simulink model "launch_sim"  (R2019a)
settings: Solver=ode4  StartTime=0.0  StopTime=20  FixedStep=.0001  RelTol=1e-3
values from neighbouring files (symbols this model uses):
  Cd = .51    (= 0.51)    [load_constants.m]
  diameter = 0.156337    [load_constants.m]
  padLat = 40.2    [load_constants.m]
  padLong = 76.8    [load_constants.m]
  propWeight = 1.2700    (= 1.27)    [motor.m]
  rocketMass = 15.51286 - totalWeight    [load_constants.m]
  thrust = thrustData(:,2)    [motor.m]
  thrustTime = thrustData(:,1)    [motor.m]
  totalImpulse = 2856.1    [motor.m]
  totalWeight = propWeight + 1.2515    (= 2.5215)    [motor.m]
libraries: simulink x3, aerolibatmos2 x1, dspstat3 x1, dspindex x1
settings Model: ExtModeTrigMode=oneshot  ExtModeArmWhenConnect=off  Creator=jkerns1  LastModifiedBy=dstum
settings DataIOCC: SaveFormat=Array  SignalLoggingSaveFormat=ModelDataLogs  ReturnWorkspaceOutputs=off
settings OptimizationCC: BlockReduction=off  BooleanDataType=off  ExpressionDepthLimit=2147483647  LifeSpan=inf
settings DebuggingCC: SaveWithParameterizedLinksMsg=none  UnderspecifiedInitializationDetection=Classic  MergeDetectMultiDrivingBlocksExec=none  SignalResolutionControl=TryResolveAllWithWarning  MultiTaskDSMMsg=warning  MultiTaskCondExecSysMsg=none  FcnCallInpInsideContextMsg=warning  StateNameClashWarn=warning  SFUnexpectedBacktrackingDiag=warning  SFNoUnconditionalDefaultTransitionDiag=warning  SFExecutionAtInitializationDiag=none  ArithmeticOperatorsInVariantConditions=warning
settings HardwareCC: ProdBitPerPointer=32  ProdBitPerSizeT=32  ProdBitPerPtrDiffT=32  ProdLargestAtomicFloat=None  ProdIntDivRoundTo=Undefined  ProdEndianess=Unspecified  ProdWordSize=32  ProdHWDeviceType=32-bit Generic  TargetUnknown=on
settings ModelReferenceCC: PropagateSignalLabelsOutOfModel=off
settings SFSimCC: SimUseLocalCustomCode=off
settings RTWCC: RTWUseLocalCustomCode=off
settings CodeAppCC: StateflowObjectComments=on
settings GRTTargetCC: TargetLangStandard=C89/C90 (ANSI)  GeneratePreprocessorConditionals=Disable all  CombineOutputUpdateFcns=off  GRTInterface=on
settings ConfigComp: CovMetricSettings=dw  CovHtmlReporting=on  CovSaveCumulativeToWorkspaceVar=on  CovSaveSingleToWorkspaceVar=on  CovExternalEMLEnable=off

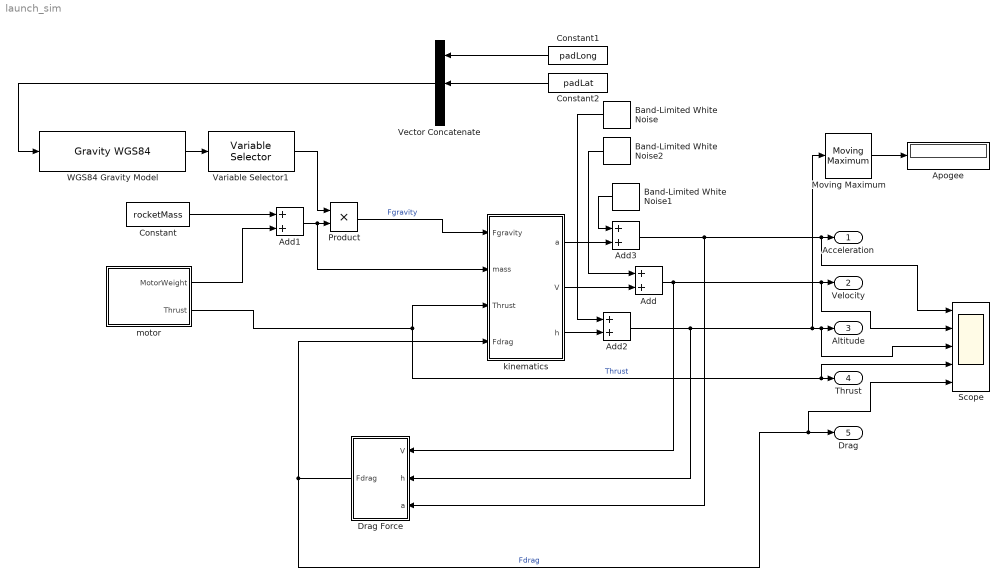
== system launch_sim ==
  Add{,1..3} (4 alike) : Sum
  Apogee : Display
  Band-Limited White Noise : simulink/Sources/Band-Limited White Noise  Cov=[.01]  Ts=0.1  seed=[23371]
  Band-Limited White Noise1 : simulink/Sources/Band-Limited White Noise  Cov=[.01]  Ts=0.1  seed=[23741]
  Band-Limited White Noise2 : simulink/Sources/Band-Limited White Noise  Cov=[.01]  Ts=0.1  seed=[23541]
  Constant : Constant  Value=rocketMass
  Constant1 : Constant  Value=padLong
  Constant2 : Constant  Value=padLat
  Drag Force : Subsystem
  Moving Maximum : dspstat3/Moving Maximum  SpecifyWindowLength=off  WindowLength=100000  SimulateUsing=Code generation
      settings: SourceProductName=DSP System Toolbox  SourceProductBaseCode=DS
  Product : Product
  Scope : Scope  NumInputPorts=5
  Variable Selector1 : dspindex/Variable Selector  NumInputs=1  rowsOrCols=Columns  IdxMode=Fixed  Elements=3  ZerOneIdxMode=One-based  errmode=Clip Index  FillMode=on  FillValues=0
  Vector Concatenate : Concatenate  NumInputs=3
  "WGS84 Gravity Model  " : GravityWGS84  no_centrifugal=off
  kinematics : Subsystem
  motor : Subsystem
  Acceleration : Outport
  Velocity : Outport  Port=2
  Altitude : Outport  Port=3
  Thrust : Outport  Port=4
  Drag : Outport  Port=5
  wires:
  Drag Force/1(Fdrag) -> kinematics/4(Fdrag), Scope/5, Drag/1  "Fdrag"
  motor/2(Thrust) -> kinematics/3("Thrust "), Scope/4, Thrust/1  "Thrust"
  motor/1(MotorWeight) -> Add1/2
  Constant/1 -> Add1/1
  Add1/1 -> kinematics/2(mass), Product/2
  Moving Maximum/1 -> Apogee/1
  Constant2/1 -> Vector Concatenate/2
  Constant1/1 -> Vector Concatenate/1
  Vector Concatenate/1 -> "WGS84 Gravity Model  "/1
  "WGS84 Gravity Model  "/1 -> Variable Selector1/1
  Variable Selector1/1 -> Product/1
  Product/1 -> kinematics/1(Fgravity)  "Fgravity"
  Band-Limited White Noise/1 -> Add2/1
  kinematics/3(h) -> Add2/2
  kinematics/2(V) -> Add/2
  kinematics/1(a) -> Add3/2
  Band-Limited White Noise1/1 -> Add3/1
  Band-Limited White Noise2/1 -> Add/1
  Add/1 -> Scope/2, Velocity/1, Drag Force/1(V)
  Add2/1 -> Drag Force/2(h), Moving Maximum/1, Scope/3, Altitude/1
  Add3/1 -> Drag Force/3(a), Scope/1, Acceleration/1

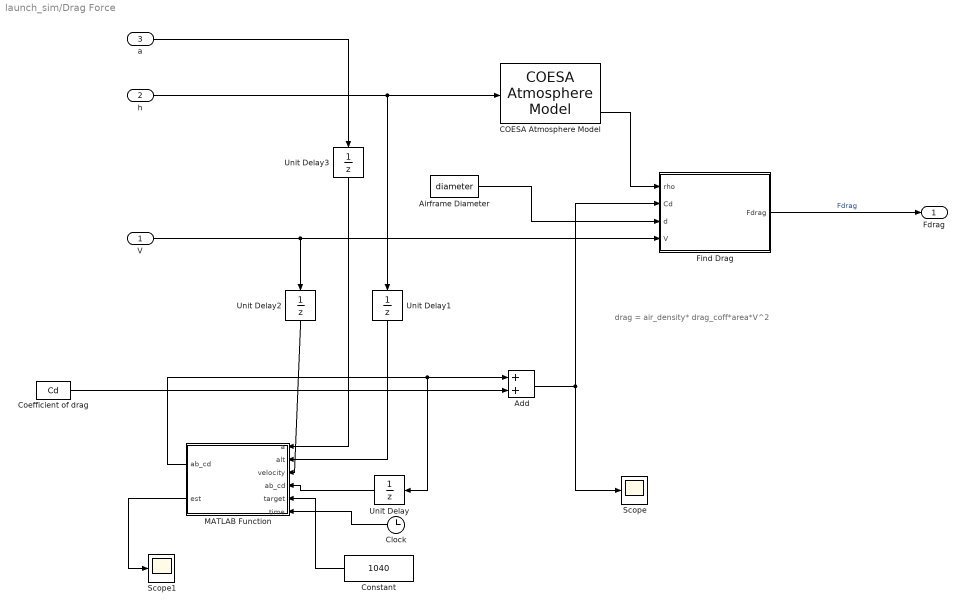
== system launch_sim/Drag Force ==
  note: drag = air_density* drag_coff*area*V^2
  V : Inport
  h : Inport  Port=2
  a : Inport  Port=3
  Add : Sum
  Airframe Diameter : Constant  Value=diameter
  COESA Atmosphere Model : aerolibatmos2/COESA Atmosphere Model  units=Metric (MKS)  spec=1976 COESA-extended U.S. Standard Atmosphere  model=Profile  profile_var=Low density  profile_percent=1%  profile_alt=5 km (16404 ft)  envelope_var=High temperature  envelope_percent=1%  action=Warning
  Clock : Clock
  Coefficient of drag : Constant  Value=Cd
  Constant : Constant  Value=1040
  Find Drag : Subsystem
  MATLAB Function : MATLAB Function  TreatAsAtomicUnit=on
  Scope : Scope
  Scope1 : Scope
  Unit Delay{,1..3} (4 alike) : UnitDelay  SampleTime=-1  HasFrameUpgradeWarning=on
  Fdrag : Outport
  wires:
  h/1 -> COESA Atmosphere Model/1, Unit Delay1/1
  Find Drag/1(Fdrag) -> Fdrag/1  "Fdrag"
  Airframe Diameter/1 -> Find Drag/3(d)
  V/1 -> Find Drag/4(V), Unit Delay2/1
  COESA Atmosphere Model/4 -> Find Drag/1(rho)
  Coefficient of drag/1 -> Add/2
  Add/1 -> Scope/1, Find Drag/2(Cd)
  Unit Delay/1 -> MATLAB Function/4("ab_cd ")
  MATLAB Function/1(ab_cd) -> Unit Delay/1, Add/1
  Unit Delay1/1 -> MATLAB Function/2(alt)
  Unit Delay2/1 -> MATLAB Function/3(velocity)
  Unit Delay3/1 -> MATLAB Function/1(a)
  a/1 -> Unit Delay3/1
  MATLAB Function/2(est) -> Scope1/1
  Constant/1 -> MATLAB Function/5(target)
  Clock/1 -> MATLAB Function/6(time)

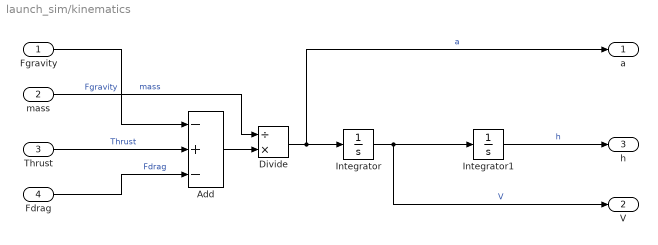
== system launch_sim/kinematics ==
  Fgravity : Inport
  mass : Inport  Port=2
  "Thrust " : Inport  Port=3
  Fdrag : Inport  Port=4
  Add : Sum  Inputs=-+-
  Divide : Product  Inputs=/*
  Integrator : Integrator
  Integrator1 : Integrator
  a : Outport
  V : Outport  Port=2
  h : Outport  Port=3
  wires:
  Divide/1 -> a/1, Integrator/1  "a"
  Fdrag/1 -> Add/3  "Fdrag"
  Add/1 -> Divide/2
  Integrator/1 -> Integrator1/1, V/1  "V"
  "Thrust "/1 -> Add/2  "Thrust"
  mass/1 -> Divide/1  "mass"
  Integrator1/1 -> h/1  "h"
  Fgravity/1 -> Add/1  "Fgravity"

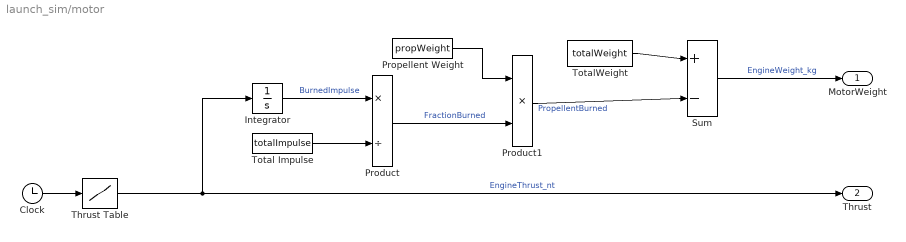
== system launch_sim/motor ==
  Clock : Clock
  Integrator : Integrator
  Product : Product  Inputs=*/  SaturateOnIntegerOverflow=on  RndMeth=Zero  InputSameDT=on  OutDataTypeStr=Inherit: Same as first input
  Product1 : Product  SaturateOnIntegerOverflow=on  RndMeth=Zero  InputSameDT=on  OutDataTypeStr=Inherit: Same as first input
  Propellent Weight : Constant  Value=propWeight
  Sum : Sum  Inputs=+|-  SaturateOnIntegerOverflow=on  InputSameDT=on  OutDataTypeStr=Inherit: Same as first input
  Thrust Table : Lookup  InputValues=thrustTime  Table=thrust  LookUpMeth=Interpolation-Use End Values  SaturateOnIntegerOverflow=on
  Total Impulse : Constant  Value=totalImpulse
  TotalWeight : Constant  Value=totalWeight
  MotorWeight : Outport
  Thrust : Outport  Port=2
  wires:
  Clock/1 -> Thrust Table/1
  Thrust Table/1 -> Integrator/1, Thrust/1  "EngineThrust_nt"
  Total Impulse/1 -> Product/2
  Propellent Weight/1 -> Product1/1
  TotalWeight/1 -> Sum/1
  Product/1 -> Product1/2  "FractionBurned"
  Integrator/1 -> Product/1  "BurnedImpulse"
  Product1/1 -> Sum/2  "PropellentBurned"
  Sum/1 -> MotorWeight/1  "EngineWeight_kg"

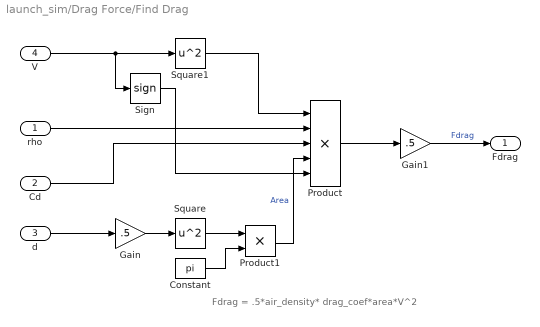
== system launch_sim/Drag Force/Find Drag ==
  note: Fdrag = .5*air_density* drag_coef*area*V^2
  rho : Inport
  Cd : Inport  Port=2
  d : Inport  Port=3
  V : Inport  Port=4
  Constant : Constant  Value=pi
  Gain : Gain  Gain=.5
  Gain1 : Gain  Gain=.5
  Product : Product  Inputs=5
  Product1 : Product
  Sign : Signum
  Square : Math  Operator=square  SaturateOnIntegerOverflow=on
  Square1 : Math  Operator=square  SaturateOnIntegerOverflow=on
  Fdrag : Outport
  wires:
  Square/1 -> Product1/1
  Constant/1 -> Product1/2
  Product1/1 -> Product/4  "Area"
  Cd/1 -> Product/3
  rho/1 -> Product/2
  d/1 -> Gain/1
  Gain/1 -> Square/1
  Product/1 -> Gain1/1
  Gain1/1 -> Fdrag/1  "Fdrag"
  V/1 -> Sign/1, Square1/1
  Square1/1 -> Product/1
  Sign/1 -> Product/5

== matlab function launch_sim/Drag Force/MATLAB Function ==
  data: a input; alt input; ab_cd output; velocity input; ab_cd input; est output; target input; time input
function [ab_cd, est]  = airbrake( a, alt, velocity, ab_cd, target, time)

est = alt + (velocity.^2)/(2*-a);

if (est) > target && time > 6
    if (ab_cd < 1.5)
        ab_cd = ab_cd + .02;
    end
elseif time > 6 && est < target
    if (ab_cd >= .2)
        
        ab_cd = ab_cd - .02;
    end
else
    ab_cd = 0;
end
